simulink model "controller"  (R2015b)
settings: Solver=FixedStepAuto  StartTime=0.0  StopTime=50  FixedStep=0.01  RelTol=1e-3
values from neighbouring files (symbols this model uses):
  aGravityCompensation = 3.5837    [controllerParams.m]
  bGravityCompensation = 2.042    [controllerParams.m]
  cGravityCompensation = 0.3    [controllerParams.m]
  D2R = pi/180.0    (= 0.0174532925199)    [controllerParams.m]
  filterCoeffs = filterCoeffs.b    [controllerParams.m]
  K_CABLE = 3    [controllerParams.m]
  K_DAQ = 10    [controllerParams.m]
  KdElev = 0    [controllerParams.m]
  KdElevRate = 0.5    [controllerParams.m]
  KdPitch = 0.3    [controllerParams.m]
  KdPitchRate = 0.2    [controllerParams.m]
  KdTrav = 0    [controllerParams.m]
  KdTravRate = 0    [controllerParams.m]
  KE_C2D = -360/4096    (= -0.087890625)    [controllerParams.m]
  KiElev = 0    [controllerParams.m]
  KiElevRate = 0.2    [controllerParams.m]
  KiPitch = 0    [controllerParams.m]
  KiPitchRate = 0.2    [controllerParams.m]
  KiTrav = 0    [controllerParams.m]
  KiTravRate = 0    [controllerParams.m]
  KpElev = 0.76    [controllerParams.m]
  KpElevRate = 5.99    [controllerParams.m]
  KpPitch = 1.11    [controllerParams.m]
  KpPitchRate = 0.78    [controllerParams.m]
  KpTrav = 0.42    [controllerParams.m]
  KpTravRate = 2.49    [controllerParams.m]
  maxDeltaForce = 0.5    [controllerParams.m]
  maxElevCombForce = 2    [controllerParams.m]
  maxElevForce = 2    [controllerParams.m]
  maxElevRate = deg2rad(20)    [controllerParams.m]
  maxIntegralElev = inf    [controllerParams.m]
  maxIntegralElevRate = inf    [controllerParams.m]
  maxIntegralPitch = inf    [controllerParams.m]
  maxIntegralPitchRate = inf    [controllerParams.m]
  maxIntegralTrav = inf    [controllerParams.m]
  maxIntegralTravRate = inf    [controllerParams.m]
  maxPitchRate = deg2rad(35)    [controllerParams.m]
  maxTravForce = 0.9    [controllerParams.m]
  maxTravRate = deg2rad(20)    [controllerParams.m]
  minDeltaForce = -0.5    [controllerParams.m]
  minElevCombForce = 0    [controllerParams.m]
  minElevForce = -2    [controllerParams.m]
  minElevRate = -deg2rad(20)    [controllerParams.m]
  minIntegralElev = -inf    [controllerParams.m]
  minIntegralElevRate = -inf    [controllerParams.m]
  minIntegralPitch = -inf    [controllerParams.m]
  minIntegralPitchRate = -inf    [controllerParams.m]
  minIntegralTrav = -inf    [controllerParams.m]
  minIntegralTravRate = -inf    [controllerParams.m]
  minPitchRate = -deg2rad(35)    [controllerParams.m]
  minTravForce = -0.9    [controllerParams.m]
  minTravRate = -deg2rad(20)    [controllerParams.m]
  tuningElevRateRef = maxElevRate    [controllerParams.m]
  tuningElevRef = deg2rad(24.5)    [controllerParams.m]
  tuningPitchRateRef = maxPitchRate    [controllerParams.m]
  tuningPitchRef = deg2rad(30)    [controllerParams.m]
  tuningTravRateRef = maxTravRate    [controllerParams.m]
  tuningTravRef = deg2rad(45)    [controllerParams.m]
  VSUM_MAX = 30    [controllerParams.m]
undefined symbols (not defined in the file or in its folder): HIL
libraries: quarc_library x6, simulink_extras x2
settings Model: SimulationMode=external  ExtModeTrigDuration=10000  Creator=AER509  LastModifiedBy=kikut
settings SolverCC: PositivePriorityOrder=on
settings RTWCC: SystemTargetFile=quarc_win64.tlc  TemplateMakefile=quarc_default_tmf  Description=QUARC Win64 Target
settings STFCustomTargetCC: GeneratePreprocessorConditionals=Use local settings  CPPClassGenCompliant=off
settings GRTTargetCC: ParMdlRefBuildCompliant=off  CompOptLevelCompliant=off  CombineOutputUpdateFcns=off  MatFileLogging=off  CPPClassGenCompliant=off  GRTInterface=on  UseToolchainInfoCompliant=off  ExtMode=on  ExtModeMexFile=quarc_comm

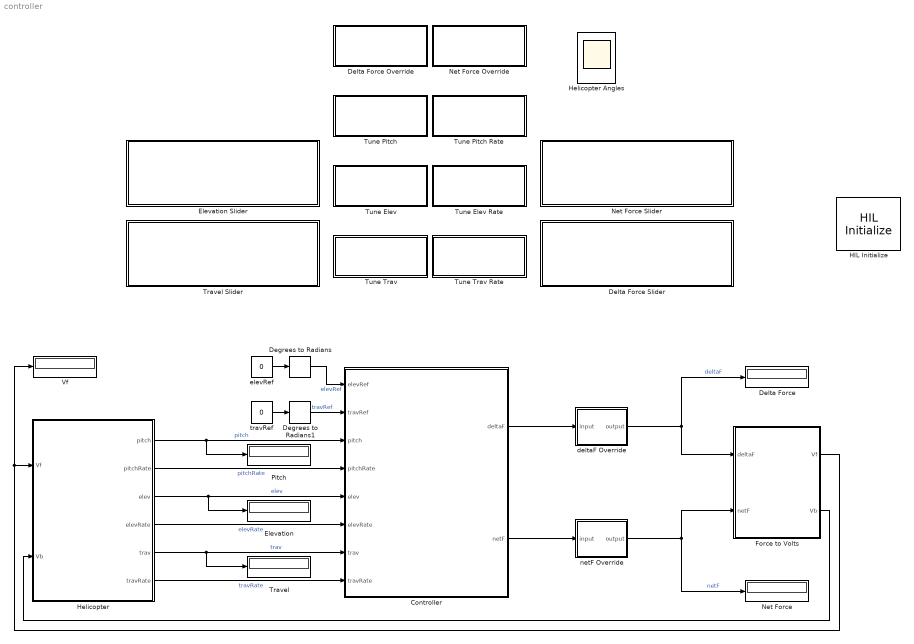
== system controller ==
  Controller : Subsystem
  Degrees to Radians : simulink_extras/Transformations/Degrees to Radians
  Degrees to Radians1 : simulink_extras/Transformations/Degrees to Radians
  Delta Force : Display
      settings: Decimation=2
  Delta Force Override : Subsystem  DialogController=hmiCreateDDGDialog  IsWebBlock=on  mask(MWDashboardBlock){webBlockId=4af075b6-758d-4f73-8e94-205a8f4b4bc9, webBlockType=sliderswitch, ShowInLibBrowser=on, ShowInitialText=on, HMISrcModelName=controller}
      mask prompts: webBlockId "WebBlock Id"; webBlockType "WebBlock Type"; HMISrcModelName "Source Model"
      mask Help: helpview([docroot '/mapfiles/simulink.map'], 'hmi_slider_switch')
      mask Display:
      | if strcmp(get_param(bdroot(gcb),'BlockDiagramType'), 'library')
      |     image([(matlabroot) '/toolbox/simulink/hmi/icons/SliderSwitch.png']);
      | end
  Delta Force Slider : Subsystem  DialogController=hmiCreateDDGDialog  IsWebBlock=on  mask(MWDashboardBlock){webBlockId=28de445a-717c-4887-bbc9-b4fa61ddbf15, webBlockType=slider, ShowInLibBrowser=on, ShowInitialText=on, HMISrcModelName=controller}
      mask prompts: webBlockId "WebBlock Id"; webBlockType "WebBlock Type"; HMISrcModelName "Source Model"
      mask Help: helpview([docroot '/mapfiles/simulink.map'], 'hmi_slider')
      mask Display:
      | if strcmp(get_param(bdroot(gcb),'BlockDiagramType'), 'library')
      |     image([(matlabroot) '/toolbox/simulink/hmi/icons/Slider.png']);
      | end
  Elevation : Display
      settings: Decimation=2
  Elevation Slider : Subsystem  DialogController=hmiCreateDDGDialog  IsWebBlock=on  mask(MWDashboardBlock){webBlockId=3dc72f43-562a-447e-a206-2819fa9ff394, webBlockType=slider, ShowInLibBrowser=on, ShowInitialText=on, HMISrcModelName=controller}
      mask prompts: webBlockId "WebBlock Id"; webBlockType "WebBlock Type"; HMISrcModelName "Source Model"
      mask Help: helpview([docroot '/mapfiles/simulink.map'], 'hmi_slider')
      mask Display:
      | if strcmp(get_param(bdroot(gcb),'BlockDiagramType'), 'library')
      |     image([(matlabroot) '/toolbox/simulink/hmi/icons/Slider.png']);
      | end
  Force to Volts : Subsystem
  HIL Initialize : quarc_library/Data Acquisition/Generic/Configuration/HIL Initialize  Priority=-99  object_name=HIL-1  board_type=q4  board_number=0  board_options=""  exclusive=off  active=off  hardware_clocks=[0:1]  clock_modes=[0 0]  initial_clock_frequencies=[]  set_clock_params_at_start=on  set_clock_params_at_switch_in=off  set_clock_frequencies_at_start=off  set_clock_frequencies_at_switch_in=off  analog_input_channels=[0:3]  analog_input_maximums=10  analog_input_minimums=-10  set_analog_input_params_at_start=off  set_analog_input_params_at_switch_in=off  analog_output_channels=[0:3]  analog_output_maximums=[10]  analog_output_minimums=[-10]  initial_analog_outputs=[0]  final_analog_outputs=[0]  watchdog_analog_outputs=0  set_analog_output_params_at_start=on  set_analog_output_params_at_switch_in=off  set_analog_outputs_at_start=on  set_analog_outputs_at_switch_in=off  set_analog_outputs_at_terminate=on  set_analog_outputs_at_switch_out=off  set_analog_outputs_on_watchdog=off  digital_input_channels=[]  digital_output_channels=[]  digital_output_configuration=[]  initial_digital_outputs=[1]  final_digital_outputs=[1]  watchdog_digital_outputs=[2]  set_digital_output_params_at_start=off  set_digital_output_params_at_switch_in=off  set_digital_outputs_at_start=on  set_digital_outputs_at_switch_in=off  set_digital_outputs_at_terminate=on  set_digital_outputs_at_switch_out=off  set_digital_outputs_on_watchdog=off  encoder_channels=[0:3]  quadrature=[4]  encoder_filter_frequency=(1/60e-9)/1  initial_encoder_counts=[0]  set_encoder_params_at_start=on  set_encoder_params_at_switch_in=off  set_encoder_counts_at_start=on  set_encoder_counts_at_switch_in=off  pwm_channels=[]  pwm_modes=[0]  pwm_frequency=(1/60e-9)/1024  pwm_configuration=[]  pwm_alignment=[]  pwm_polarity=[]  pwm_leading_deadband=[]  pwm_trailing_deadband=[]  initial_pwm_outputs=[0]  final_pwm_outputs=[0]  watchdog_pwm_outputs=[]  set_pwm_params_at_start=on  set_pwm_params_at_switch_in=off  set_pwm_outputs_at_start=on  set_pwm_outputs_at_switch_in=off  set_pwm_outputs_at_terminate=on  set_pwm_outputs_at_switch_out=off  set_pwm_outputs_on_watchdog=off  other_output_channels=[]  initial_other_outputs=[]  final_other_outputs=[]  watchdog_other_outputs=[]  set_other_outputs_at_start=off  set_other_outputs_at_switch_in=off  set_other_outputs_at_terminate=off  set_other_outputs_at_switch_out=off  set_other_outputs_on_watchdog=off
  Helicopter : Subsystem
  Helicopter Angles : Scope
      settings: Floating=on
  Net Force : Display
      settings: Decimation=2
  Net Force Override : Subsystem  DialogController=hmiCreateDDGDialog  IsWebBlock=on  mask(MWDashboardBlock){webBlockId=fdba1945-908f-46ed-bc95-797a072fabde, webBlockType=sliderswitch, ShowInLibBrowser=on, ShowInitialText=on, HMISrcModelName=controller}
      mask prompts: webBlockId "WebBlock Id"; webBlockType "WebBlock Type"; HMISrcModelName "Source Model"
      mask Help: helpview([docroot '/mapfiles/simulink.map'], 'hmi_slider_switch')
      mask Display:
      | if strcmp(get_param(bdroot(gcb),'BlockDiagramType'), 'library')
      |     image([(matlabroot) '/toolbox/simulink/hmi/icons/SliderSwitch.png']);
      | end
  Net Force Slider : Subsystem  DialogController=hmiCreateDDGDialog  IsWebBlock=on  mask(MWDashboardBlock){webBlockId=5aa08be6-65a4-4742-946a-0d5b8d80040d, webBlockType=slider, ShowInLibBrowser=on, ShowInitialText=on, HMISrcModelName=controller}
      mask prompts: webBlockId "WebBlock Id"; webBlockType "WebBlock Type"; HMISrcModelName "Source Model"
      mask Help: helpview([docroot '/mapfiles/simulink.map'], 'hmi_slider')
      mask Display:
      | if strcmp(get_param(bdroot(gcb),'BlockDiagramType'), 'library')
      |     image([(matlabroot) '/toolbox/simulink/hmi/icons/Slider.png']);
      | end
  Pitch : Display
      settings: Decimation=2
  Travel : Display
      settings: Decimation=2
  Travel Slider : Subsystem  DialogController=hmiCreateDDGDialog  IsWebBlock=on  mask(MWDashboardBlock){webBlockId=229cecbd-6c7e-45e2-a8fb-f334730ec9ad, webBlockType=slider, ShowInLibBrowser=on, ShowInitialText=on, HMISrcModelName=controller}
      mask prompts: webBlockId "WebBlock Id"; webBlockType "WebBlock Type"; HMISrcModelName "Source Model"
      mask Help: helpview([docroot '/mapfiles/simulink.map'], 'hmi_slider')
      mask Display:
      | if strcmp(get_param(bdroot(gcb),'BlockDiagramType'), 'library')
      |     image([(matlabroot) '/toolbox/simulink/hmi/icons/Slider.png']);
      | end
  Tune Elev : Subsystem  DialogController=hmiCreateDDGDialog  IsWebBlock=on  mask(MWDashboardBlock){webBlockId=e4a3f78e-3c07-4c1a-9f36-b612ed18eb99, webBlockType=sliderswitch, ShowInLibBrowser=on, ShowInitialText=on, HMISrcModelName=controller}
      mask prompts: webBlockId "WebBlock Id"; webBlockType "WebBlock Type"; HMISrcModelName "Source Model"
      mask Help: helpview([docroot '/mapfiles/simulink.map'], 'hmi_slider_switch')
      mask Display:
      | if strcmp(get_param(bdroot(gcb),'BlockDiagramType'), 'library')
      |     image([(matlabroot) '/toolbox/simulink/hmi/icons/SliderSwitch.png']);
      | end
  Tune Elev Rate : Subsystem  DialogController=hmiCreateDDGDialog  IsWebBlock=on  mask(MWDashboardBlock){webBlockId=5ad47bd1-198b-4ce9-a72d-63eab8823736, webBlockType=sliderswitch, ShowInLibBrowser=on, ShowInitialText=on, HMISrcModelName=controller}
      mask prompts: webBlockId "WebBlock Id"; webBlockType "WebBlock Type"; HMISrcModelName "Source Model"
      mask Help: helpview([docroot '/mapfiles/simulink.map'], 'hmi_slider_switch')
      mask Display:
      | if strcmp(get_param(bdroot(gcb),'BlockDiagramType'), 'library')
      |     image([(matlabroot) '/toolbox/simulink/hmi/icons/SliderSwitch.png']);
      | end
  Tune Pitch : Subsystem  DialogController=hmiCreateDDGDialog  IsWebBlock=on  mask(MWDashboardBlock){webBlockId=75521f76-8e1d-4ba6-a9fe-27f99e38a80e, webBlockType=sliderswitch, ShowInLibBrowser=on, ShowInitialText=on, HMISrcModelName=controller}
      mask prompts: webBlockId "WebBlock Id"; webBlockType "WebBlock Type"; HMISrcModelName "Source Model"
      mask Help: helpview([docroot '/mapfiles/simulink.map'], 'hmi_slider_switch')
      mask Display:
      | if strcmp(get_param(bdroot(gcb),'BlockDiagramType'), 'library')
      |     image([(matlabroot) '/toolbox/simulink/hmi/icons/SliderSwitch.png']);
      | end
  Tune Pitch Rate : Subsystem  DialogController=hmiCreateDDGDialog  IsWebBlock=on  mask(MWDashboardBlock){webBlockId=8d4346d9-8b28-4eb4-a156-b2d2519f8294, webBlockType=sliderswitch, ShowInLibBrowser=on, ShowInitialText=on, HMISrcModelName=controller}
      mask prompts: webBlockId "WebBlock Id"; webBlockType "WebBlock Type"; HMISrcModelName "Source Model"
      mask Help: helpview([docroot '/mapfiles/simulink.map'], 'hmi_slider_switch')
      mask Display:
      | if strcmp(get_param(bdroot(gcb),'BlockDiagramType'), 'library')
      |     image([(matlabroot) '/toolbox/simulink/hmi/icons/SliderSwitch.png']);
      | end
  Tune Trav : Subsystem  DialogController=hmiCreateDDGDialog  IsWebBlock=on  mask(MWDashboardBlock){webBlockId=cd129c28-8443-4f24-80a9-9a0e47c4c0a7, webBlockType=sliderswitch, ShowInLibBrowser=on, ShowInitialText=on, HMISrcModelName=controller}
      mask prompts: webBlockId "WebBlock Id"; webBlockType "WebBlock Type"; HMISrcModelName "Source Model"
      mask Help: helpview([docroot '/mapfiles/simulink.map'], 'hmi_slider_switch')
      mask Display:
      | if strcmp(get_param(bdroot(gcb),'BlockDiagramType'), 'library')
      |     image([(matlabroot) '/toolbox/simulink/hmi/icons/SliderSwitch.png']);
      | end
  Tune Trav Rate : Subsystem  DialogController=hmiCreateDDGDialog  IsWebBlock=on  mask(MWDashboardBlock){webBlockId=cd69dbce-f23b-4e1a-b675-1ecb4e30d85c, webBlockType=sliderswitch, ShowInLibBrowser=on, ShowInitialText=on, HMISrcModelName=controller}
      mask prompts: webBlockId "WebBlock Id"; webBlockType "WebBlock Type"; HMISrcModelName "Source Model"
      mask Help: helpview([docroot '/mapfiles/simulink.map'], 'hmi_slider_switch')
      mask Display:
      | if strcmp(get_param(bdroot(gcb),'BlockDiagramType'), 'library')
      |     image([(matlabroot) '/toolbox/simulink/hmi/icons/SliderSwitch.png']);
      | end
  Vf : Display
      settings: Decimation=2
  deltaF Override : Subsystem
  elevRef : Constant  Value=0
  netF Override : Subsystem
  travRef : Constant  Value=0
  wires:
  Helicopter/1(pitch) -> Pitch/1, Controller/3(pitch)  "pitch"
  Helicopter/2(pitchRate) -> Controller/4(pitchRate)  "pitchRate"
  Helicopter/3(elev) -> Elevation/1, Controller/5(elev)  "elev"
  Helicopter/4(elevRate) -> Controller/6(elevRate)  "elevRate"
  Helicopter/5(trav) -> Travel/1, Controller/7(trav)  "trav"
  Helicopter/6(travRate) -> Controller/8(travRate)  "travRate"
  Controller/2(netF) -> netF Override/1(input)
  netF Override/1(output) -> Net Force/1, Force to Volts/2(netF)  "netF"
  Controller/1(deltaF) -> deltaF Override/1(input)
  deltaF Override/1(output) -> Delta Force/1, Force to Volts/1(deltaF)  "deltaF"
  elevRef/1 -> Degrees to Radians/1
  travRef/1 -> Degrees to Radians1/1
  Degrees to Radians/1 -> Controller/1(elevRef)  "elevRef"
  Degrees to Radians1/1 -> Controller/2(travRef)  "travRef"
  Force to Volts/2(Vb) -> Helicopter/2(Vb)
  Force to Volts/1(Vf) -> Vf/1, Helicopter/1(Vf)

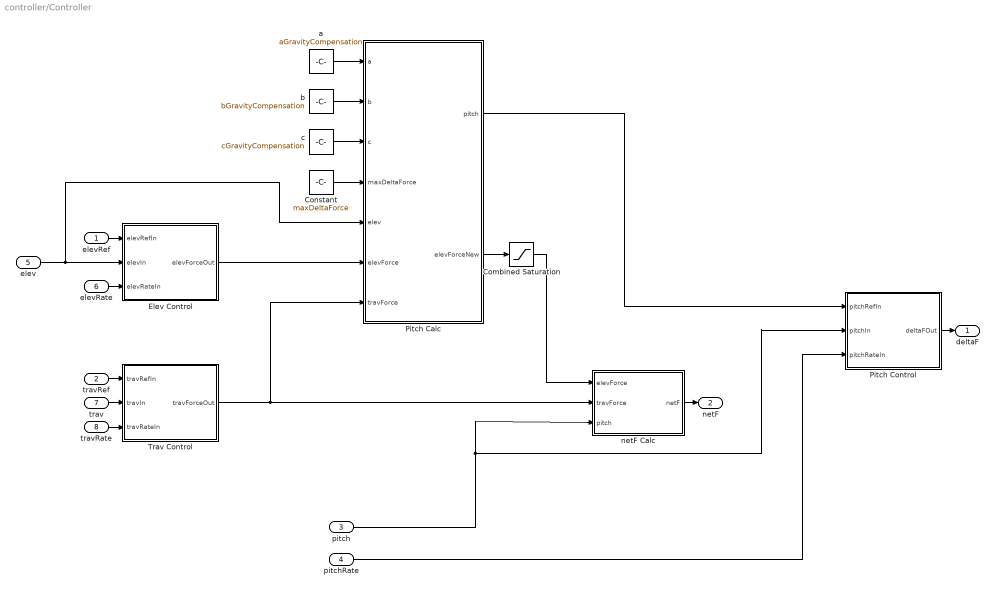
== system controller/Controller ==
  elevRef : Inport
  travRef : Inport  Port=2
  pitch : Inport  Port=3
  pitchRate : Inport  Port=4
  elev : Inport  Port=5
  elevRate : Inport  Port=6
  trav : Inport  Port=7
  travRate : Inport  Port=8
  Combined Saturation : Saturate  UpperLimit=maxElevCombForce  LowerLimit=minElevCombForce
  Constant : Constant  Value=maxDeltaForce
  Elev Control : Subsystem
  Pitch Calc : MATLAB Function  TreatAsAtomicUnit=on
  Pitch Control : Subsystem
  Trav Control : Subsystem
  a : Constant  Value=aGravityCompensation
  b : Constant  Value=bGravityCompensation
  c : Constant  Value=cGravityCompensation
  netF Calc : MATLAB Function  TreatAsAtomicUnit=on
  deltaF : Outport
  netF : Outport  Port=2
  wires:
  Trav Control/1(travForceOut) -> Pitch Calc/7(travForce), netF Calc/2(travForce)
  Elev Control/1(elevForceOut) -> Pitch Calc/6(elevForce)
  pitchRate/1 -> Pitch Control/3(pitchRateIn)
  netF Calc/1(netF) -> netF/1
  elev/1 -> Pitch Calc/5(elev), Elev Control/2(elevIn)
  elevRate/1 -> Elev Control/3(elevRateIn)
  elevRef/1 -> Elev Control/1(elevRefIn)
  Pitch Control/1(deltaFOut) -> deltaF/1
  Pitch Calc/2(elevForceNew) -> Combined Saturation/1
  travRate/1 -> Trav Control/3(travRateIn)
  trav/1 -> Trav Control/2(travIn)
  travRef/1 -> Trav Control/1(travRefIn)
  Pitch Calc/1(pitch) -> Pitch Control/1(pitchRefIn)
  pitch/1 -> netF Calc/3(pitch), Pitch Control/2(pitchIn)
  Constant/1 -> Pitch Calc/4(maxDeltaForce)
  Combined Saturation/1 -> netF Calc/1(elevForce)
  a/1 -> Pitch Calc/1(a)
  b/1 -> Pitch Calc/2(b)
  c/1 -> Pitch Calc/3(c)

== system controller/Delta Force Override ==

== system controller/Delta Force Slider ==

== system controller/Elevation Slider ==

== system controller/Force to Volts ==
  deltaF : Inport
  netF : Inport  Port=2
  Force Mixer : MATLAB Function  TreatAsAtomicUnit=on
  Force to Volt_Back : MATLAB Function  TreatAsAtomicUnit=on
  Force to Volt_Front : MATLAB Function  TreatAsAtomicUnit=on
  Vf : Outport
  Vb : Outport  Port=2
  wires:
  Force Mixer/1(F_f) -> Force to Volt_Front/1(F)
  Force to Volt_Front/1(V) -> Vf/1  "V_f"
  Force Mixer/2(F_b) -> Force to Volt_Back/1(F)
  Force to Volt_Back/1(V) -> Vb/1  "V_b"
  netF/1 -> Force Mixer/2(F)
  deltaF/1 -> Force Mixer/1(delta_F)

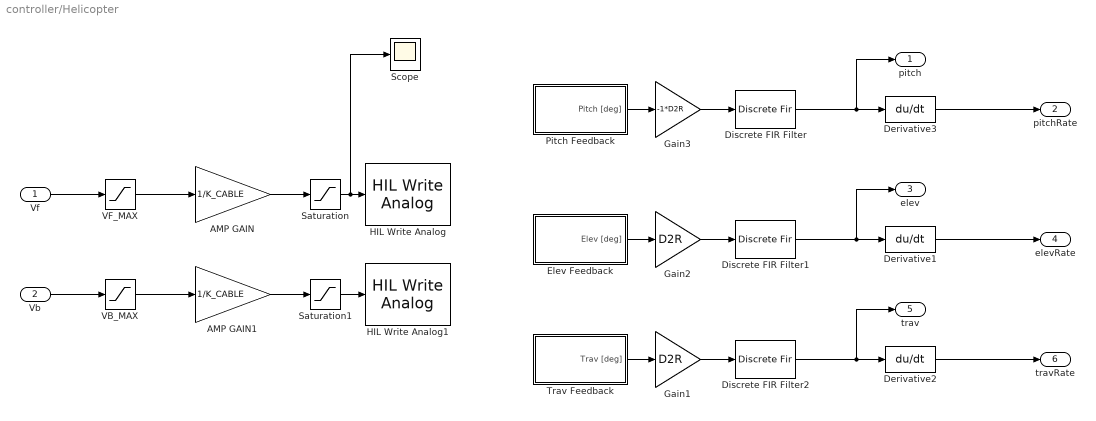
== system controller/Helicopter ==
  Vf : Inport
  Vb : Inport  Port=2
  AMP GAIN : Gain  Gain=1/K_CABLE
  AMP GAIN1 : Gain  Gain=1/K_CABLE
  Derivative1 : Derivative
  Derivative2 : Derivative
  Derivative3 : Derivative
  Discrete FIR Filter : DiscreteFir  Coefficients=filterCoeffs
  Discrete FIR Filter1 : DiscreteFir  Coefficients=filterCoeffs
  Discrete FIR Filter2 : DiscreteFir  Coefficients=filterCoeffs
  Elev Feedback : Subsystem
  Gain1 : Gain  Gain=D2R
  Gain2 : Gain  Gain=D2R
  Gain3 : Gain  Gain=-1*D2R
  HIL Write Analog : quarc_library/Data Acquisition/Generic/Immediate I//O/HIL Write Analog  object_name=HIL-1  channels=2  sample_time=-1  active=off  vector_input=off
  HIL Write Analog1 : quarc_library/Data Acquisition/Generic/Immediate I//O/HIL Write Analog  object_name=HIL-1  channels=3  sample_time=-1  active=off  vector_input=off
  Pitch Feedback : Subsystem
  Saturation : Saturate  UpperLimit=K_DAQ*0.5  LowerLimit=-K_DAQ*0.5
  Saturation1 : Saturate  UpperLimit=K_DAQ*0.5  LowerLimit=-K_DAQ*0.5
  Scope : Scope
  Trav Feedback : Subsystem
  VB_MAX : Saturate  UpperLimit=VSUM_MAX*0.5  LowerLimit=-VSUM_MAX*0.5
  VF_MAX : Saturate  UpperLimit=VSUM_MAX*0.5  LowerLimit=-VSUM_MAX*0.5  LinearizeAsGain=off
  pitch : Outport
  pitchRate : Outport  Port=2
  elev : Outport  Port=3
  elevRate : Outport  Port=4
  trav : Outport  Port=5
  travRate : Outport  Port=6
  wires:
  VB_MAX/1 -> AMP GAIN1/1
  Pitch Feedback/1(Pitch [deg]) -> Gain3/1
  Trav Feedback/1(Trav [deg]) -> Gain1/1
  Gain3/1 -> Discrete FIR Filter/1
  Saturation/1 -> Scope/1, HIL Write Analog/1
  Vf/1 -> VF_MAX/1
  VF_MAX/1 -> AMP GAIN/1
  AMP GAIN/1 -> Saturation/1
  Saturation1/1 -> HIL Write Analog1/1
  Discrete FIR Filter/1 -> pitch/1, Derivative3/1
  AMP GAIN1/1 -> Saturation1/1
  Elev Feedback/1(Elev [deg]) -> Gain2/1
  Vb/1 -> VB_MAX/1
  Derivative3/1 -> pitchRate/1
  Gain2/1 -> Discrete FIR Filter1/1
  Discrete FIR Filter1/1 -> elev/1, Derivative1/1
  Derivative1/1 -> elevRate/1
  Gain1/1 -> Discrete FIR Filter2/1
  Discrete FIR Filter2/1 -> trav/1, Derivative2/1
  Derivative2/1 -> travRate/1

== system controller/Net Force Override ==

== system controller/Net Force Slider ==

== system controller/Travel Slider ==

== system controller/Tune Elev ==

== system controller/Tune Elev Rate ==

== system controller/Tune Pitch ==

== system controller/Tune Pitch Rate ==

== system controller/Tune Trav ==

== system controller/Tune Trav Rate ==

== system controller/deltaF Override ==
  input : Inport
  Tune Selector : Subsystem
  tuneRef : Constant  Value=0
  output : Outport
  wires:
  tuneRef/1 -> Tune Selector/1(tuneRef)
  input/1 -> Tune Selector/2(defaultRef)
  Tune Selector/1("output ") -> output/1

== system controller/netF Override ==
  input : Inport
  Tune Selector : Subsystem
  tuneRef : Constant  Value=0.5875
  output : Outport
  wires:
  tuneRef/1 -> Tune Selector/1(tuneRef)
  input/1 -> Tune Selector/2(defaultRef)
  Tune Selector/1("output ") -> output/1

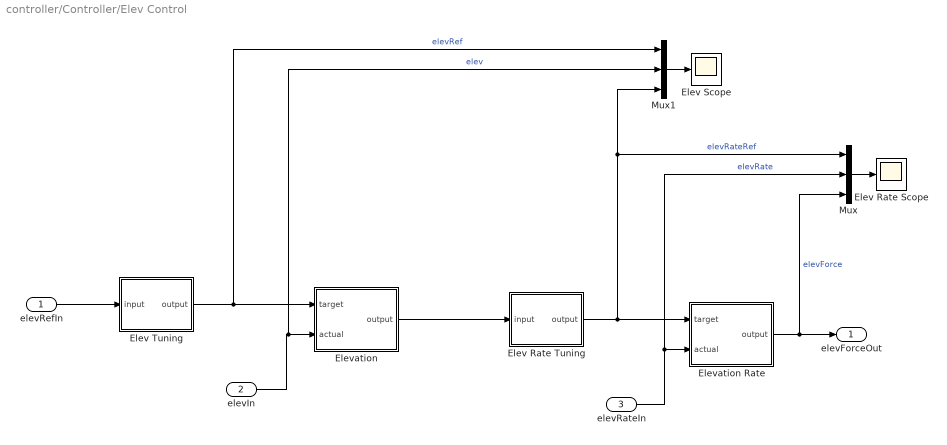
== system controller/Controller/Elev Control ==
  elevRefIn : Inport
  elevIn : Inport  Port=2
  elevRateIn : Inport  Port=3
  Elev Rate Scope : Scope
  Elev Rate Tuning : Subsystem
  Elev Scope : Scope
  Elev Tuning : Subsystem
  Elevation : Subsystem
  Elevation Rate : Subsystem
  Mux : Mux  Inputs=3
  Mux1 : Mux  Inputs=3
  elevForceOut : Outport
  wires:
  Elev Tuning/1(output) -> Mux1/1, Elevation/1(target)  "elevRef"
  Elev Rate Tuning/1(output) -> Mux1/3, Mux/1, Elevation Rate/1(target)  "elevRateRef"
  Elevation/1(output) -> Elev Rate Tuning/1(input)
  Elevation Rate/1(output) -> Mux/3, elevForceOut/1  "elevForce"
  elevRefIn/1 -> Elev Tuning/1(input)
  elevIn/1 -> Mux1/2, Elevation/2(actual)  "elev"
  elevRateIn/1 -> Mux/2, Elevation Rate/2(actual)  "elevRate"
  Mux/1 -> Elev Rate Scope/1
  Mux1/1 -> Elev Scope/1

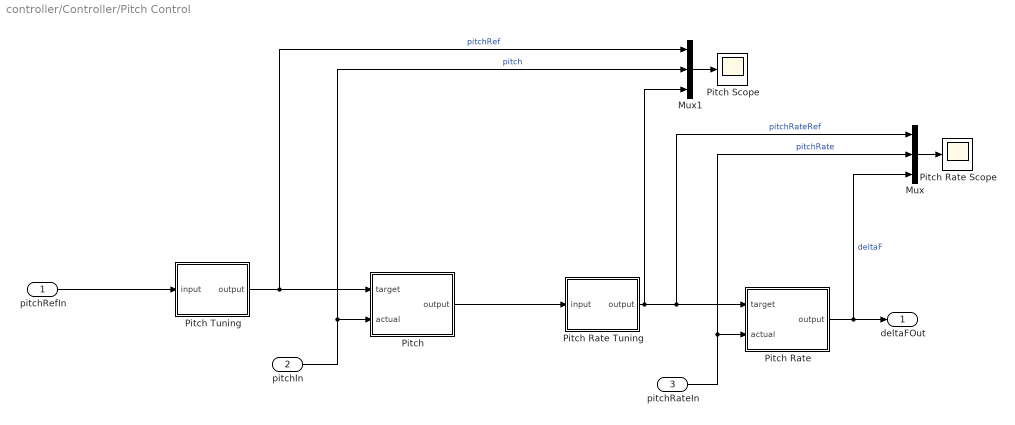
== system controller/Controller/Pitch Control ==
  pitchRefIn : Inport
  pitchIn : Inport  Port=2
  pitchRateIn : Inport  Port=3
  Mux : Mux  Inputs=3
  Mux1 : Mux  Inputs=3
  Pitch : Subsystem
  Pitch Rate : Subsystem
  Pitch Rate Scope : Scope
  Pitch Rate Tuning : Subsystem
  Pitch Scope : Scope
  Pitch Tuning : Subsystem
  deltaFOut : Outport
  wires:
  Pitch Rate/1(output) -> Mux/3, deltaFOut/1  "deltaF"
  pitchIn/1 -> Mux1/2, Pitch/2(actual)  "pitch"
  pitchRefIn/1 -> Pitch Tuning/1(input)
  Pitch Rate Tuning/1(output) -> Mux1/3, Mux/1, Pitch Rate/1(target)  "pitchRateRef"
  Pitch Tuning/1(output) -> Mux1/1, Pitch/1(target)  "pitchRef"
  Pitch/1(output) -> Pitch Rate Tuning/1(input)
  pitchRateIn/1 -> Mux/2, Pitch Rate/2(actual)  "pitchRate"
  Mux/1 -> Pitch Rate Scope/1
  Mux1/1 -> Pitch Scope/1

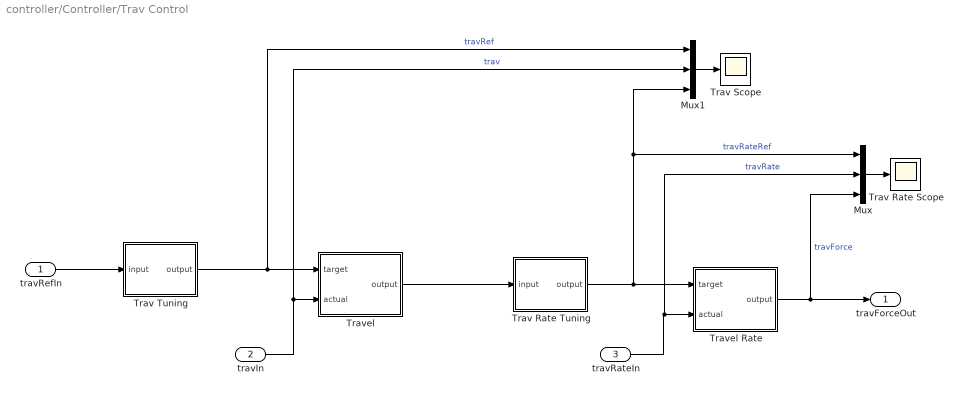
== system controller/Controller/Trav Control ==
  travRefIn : Inport
  travIn : Inport  Port=2
  travRateIn : Inport  Port=3
  Mux : Mux  Inputs=3
  Mux1 : Mux  Inputs=3
  Trav Rate Scope : Scope
  Trav Rate Tuning : Subsystem
  Trav Scope : Scope
  Trav Tuning : Subsystem
  Travel : Subsystem
  Travel Rate : Subsystem
  travForceOut : Outport
  wires:
  Travel Rate/1(output) -> Mux/3, travForceOut/1  "travForce"
  travRateIn/1 -> Mux/2, Travel Rate/2(actual)  "travRate"
  travIn/1 -> Mux1/2, Travel/2(actual)  "trav"
  travRefIn/1 -> Trav Tuning/1(input)
  Trav Tuning/1(output) -> Mux1/1, Travel/1(target)  "travRef"
  Travel/1(output) -> Trav Rate Tuning/1(input)
  Trav Rate Tuning/1(output) -> Mux1/3, Mux/1, Travel Rate/1(target)  "travRateRef"
  Mux/1 -> Trav Rate Scope/1
  Mux1/1 -> Trav Scope/1

== system controller/Helicopter/Elev Feedback ==
  Bias : Bias
  Count2Degree : Gain  Gain=KE_C2D
  HIL Read Encoder : quarc_library/Data Acquisition/Generic/Immediate I//O/HIL Read Encoder  object_name=HIL-1  channels=3  sample_time=qc_get_step_size  active=on  vector_output=off  data_type_mode=Inherit via back propagation  data_type=double
  Elev [deg] : Outport
  wires:
  Count2Degree/1 -> Bias/1
  Bias/1 -> Elev [deg]/1
  HIL Read Encoder/1 -> Count2Degree/1

== system controller/Helicopter/Pitch Feedback ==
  Bias : Bias
  Count2Degree : Gain  Gain=KE_C2D*0.5
  HIL Read Encoder : quarc_library/Data Acquisition/Generic/Immediate I//O/HIL Read Encoder  object_name=HIL-1  channels=2  sample_time=qc_get_step_size  active=on  vector_output=off  data_type_mode=Inherit via back propagation  data_type=double
  Pitch [deg] : Outport
  wires:
  Count2Degree/1 -> Bias/1
  Bias/1 -> Pitch [deg]/1
  HIL Read Encoder/1 -> Count2Degree/1

== system controller/Helicopter/Trav Feedback ==
  Bias : Bias
  Count2Degree : Gain  Gain=KE_C2D*0.5
  HIL Read Encoder : quarc_library/Data Acquisition/Generic/Immediate I//O/HIL Read Encoder  object_name=HIL-1  channels=1  sample_time=qc_get_step_size  active=on  vector_output=off  data_type_mode=Inherit via back propagation  data_type=double
  Trav [deg] : Outport
  wires:
  Count2Degree/1 -> Bias/1
  Bias/1 -> Trav [deg]/1
  HIL Read Encoder/1 -> Count2Degree/1

== system controller/deltaF Override/Tune Selector ==
  tuneRef : Inport
  defaultRef : Inport  Port=2
  Multiport Switch : MultiPortSwitch  DataPortOrder=Zero-based contiguous  Inputs=2
  deltaF : Constant  Value=0
  "output " : Outport
  wires:
  deltaF/1 -> Multiport Switch/1
  defaultRef/1 -> Multiport Switch/2
  Multiport Switch/1 -> "output "/1
  tuneRef/1 -> Multiport Switch/3

== system controller/netF Override/Tune Selector ==
  tuneRef : Inport
  defaultRef : Inport  Port=2
  Multiport Switch : MultiPortSwitch  DataPortOrder=Zero-based contiguous  Inputs=2  DataPortIndices={1,2}
  netF : Constant  Value=0
  "output " : Outport
  wires:
  netF/1 -> Multiport Switch/1
  defaultRef/1 -> Multiport Switch/2
  Multiport Switch/1 -> "output "/1
  tuneRef/1 -> Multiport Switch/3

== system controller/Controller/Elev Control/Elev Rate Tuning ==
  input : Inport
  Step : Step  Time=2  After=tuningElevRateRef  SampleTime=0
  Tune Selector : Subsystem
  output : Outport
  wires:
  Step/1 -> Tune Selector/1(tuneRef)
  input/1 -> Tune Selector/2(defaultRef)
  Tune Selector/1("output ") -> output/1

== system controller/Controller/Elev Control/Elev Tuning ==
  input : Inport
  Step : Step  Time=2  After=tuningElevRef  SampleTime=0
  Tune Selector : Subsystem
  output : Outport
  wires:
  Step/1 -> Tune Selector/1(tuneRef)
  input/1 -> Tune Selector/2(defaultRef)
  Tune Selector/1("output ") -> output/1

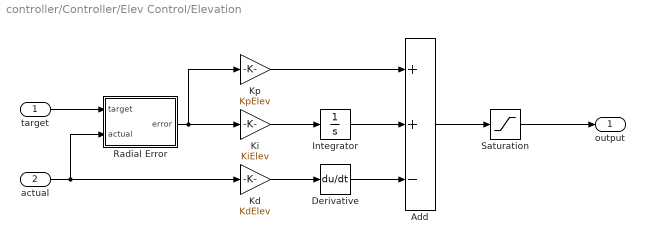
== system controller/Controller/Elev Control/Elevation ==
  target : Inport
  actual : Inport  Port=2
  Add : Sum  Inputs=++-
  Derivative : Derivative
  Integrator : Integrator  LimitOutput=on  UpperSaturationLimit=maxIntegralElev  LowerSaturationLimit=minIntegralElev
  Kd : Gain  Gain=KdElev
  Ki : Gain  Gain=KiElev
  Kp : Gain  Gain=KpElev
  Radial Error : MATLAB Function  TreatAsAtomicUnit=on
  Saturation : Saturate  UpperLimit=maxElevRate  LowerLimit=minElevRate
  output : Outport
  wires:
  Radial Error/1(error) -> Kp/1, Ki/1
  actual/1 -> Radial Error/2(actual), Kd/1
  Kd/1 -> Derivative/1
  Kp/1 -> Add/1
  Add/1 -> Saturation/1
  Integrator/1 -> Add/2
  target/1 -> Radial Error/1(target)
  Saturation/1 -> output/1
  Derivative/1 -> Add/3
  Ki/1 -> Integrator/1

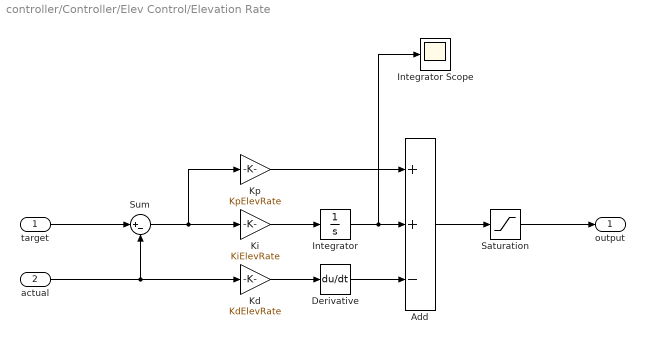
== system controller/Controller/Elev Control/Elevation Rate ==
  target : Inport
  actual : Inport  Port=2
  Add : Sum  Inputs=++-
  Derivative : Derivative
  Integrator : Integrator  LimitOutput=on  UpperSaturationLimit=maxIntegralElevRate  LowerSaturationLimit=minIntegralElevRate
  Integrator Scope : Scope
  Kd : Gain  Gain=KdElevRate
  Ki : Gain  Gain=KiElevRate
  Kp : Gain  Gain=KpElevRate
  Saturation : Saturate  UpperLimit=maxElevForce  LowerLimit=minElevForce
  Sum : Sum  Inputs=|+-
  output : Outport
  wires:
  Sum/1 -> Kp/1, Ki/1
  actual/1 -> Sum/2, Kd/1
  Kd/1 -> Derivative/1
  Kp/1 -> Add/1
  Add/1 -> Saturation/1
  Integrator/1 -> Integrator Scope/1, Add/2
  target/1 -> Sum/1
  Saturation/1 -> output/1
  Derivative/1 -> Add/3
  Ki/1 -> Integrator/1

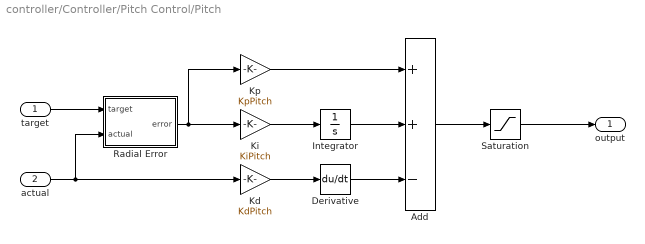
== system controller/Controller/Pitch Control/Pitch ==
  target : Inport
  actual : Inport  Port=2
  Add : Sum  Inputs=++-
  Derivative : Derivative
  Integrator : Integrator  LimitOutput=on  UpperSaturationLimit=maxIntegralPitch  LowerSaturationLimit=minIntegralPitch
  Kd : Gain  Gain=KdPitch
  Ki : Gain  Gain=KiPitch
  Kp : Gain  Gain=KpPitch
  Radial Error : MATLAB Function  TreatAsAtomicUnit=on
  Saturation : Saturate  UpperLimit=maxPitchRate  LowerLimit=minPitchRate
  output : Outport
  wires:
  Radial Error/1(error) -> Kp/1, Ki/1
  actual/1 -> Radial Error/2(actual), Kd/1
  Kd/1 -> Derivative/1
  Kp/1 -> Add/1
  Add/1 -> Saturation/1
  Integrator/1 -> Add/2
  target/1 -> Radial Error/1(target)
  Saturation/1 -> output/1
  Derivative/1 -> Add/3
  Ki/1 -> Integrator/1

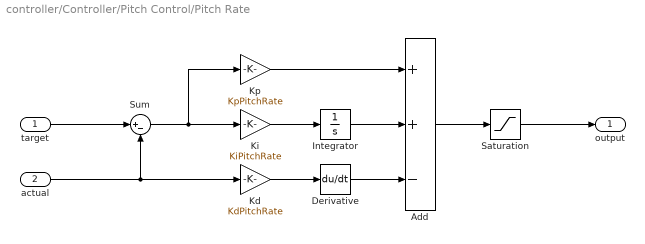
== system controller/Controller/Pitch Control/Pitch Rate ==
  target : Inport
  actual : Inport  Port=2
  Add : Sum  Inputs=++-
  Derivative : Derivative
  Integrator : Integrator  LimitOutput=on  UpperSaturationLimit=maxIntegralPitchRate  LowerSaturationLimit=minIntegralPitchRate
  Kd : Gain  Gain=KdPitchRate
  Ki : Gain  Gain=KiPitchRate
  Kp : Gain  Gain=KpPitchRate
  Saturation : Saturate  UpperLimit=maxDeltaForce  LowerLimit=minDeltaForce
  Sum : Sum  Inputs=|+-
  output : Outport
  wires:
  Sum/1 -> Kp/1, Ki/1
  actual/1 -> Sum/2, Kd/1
  Kd/1 -> Derivative/1
  Kp/1 -> Add/1
  Add/1 -> Saturation/1
  Integrator/1 -> Add/2
  target/1 -> Sum/1
  Saturation/1 -> output/1
  Derivative/1 -> Add/3
  Ki/1 -> Integrator/1

== system controller/Controller/Pitch Control/Pitch Rate Tuning ==
  input : Inport
  Step : Step  Time=2  After=tuningPitchRateRef  SampleTime=0
  Tune Selector : Subsystem
  output : Outport
  wires:
  Step/1 -> Tune Selector/1(tuneRef)
  input/1 -> Tune Selector/2(defaultRef)
  Tune Selector/1("output ") -> output/1

== system controller/Controller/Pitch Control/Pitch Tuning ==
  input : Inport
  Step : Step  Time=2  After=tuningPitchRef  SampleTime=0
  Tune Selector : Subsystem
  output : Outport
  wires:
  Step/1 -> Tune Selector/1(tuneRef)
  input/1 -> Tune Selector/2(defaultRef)
  Tune Selector/1("output ") -> output/1

== system controller/Controller/Trav Control/Trav Rate Tuning ==
  input : Inport
  Step : Step  Time=10  After=tuningTravRateRef  SampleTime=0
  Tune Selector : Subsystem
  output : Outport
  wires:
  Step/1 -> Tune Selector/1(tuneRef)
  input/1 -> Tune Selector/2(defaultRef)
  Tune Selector/1("output ") -> output/1

== system controller/Controller/Trav Control/Trav Tuning ==
  input : Inport
  Step : Step  Time=10  After=tuningTravRef  SampleTime=0
  Tune Selector : Subsystem
  output : Outport
  wires:
  Step/1 -> Tune Selector/1(tuneRef)
  input/1 -> Tune Selector/2(defaultRef)
  Tune Selector/1("output ") -> output/1

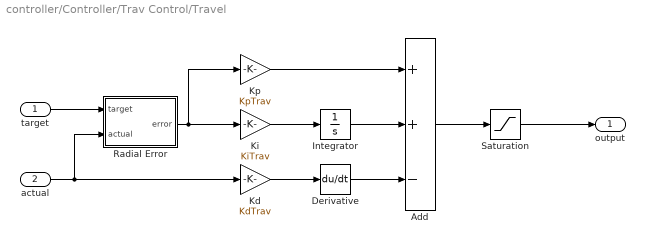
== system controller/Controller/Trav Control/Travel ==
  target : Inport
  actual : Inport  Port=2
  Add : Sum  Inputs=++-
  Derivative : Derivative
  Integrator : Integrator  LimitOutput=on  UpperSaturationLimit=maxIntegralTrav  LowerSaturationLimit=minIntegralTrav
  Kd : Gain  Gain=KdTrav
  Ki : Gain  Gain=KiTrav
  Kp : Gain  Gain=KpTrav
  Radial Error : MATLAB Function  TreatAsAtomicUnit=on
  Saturation : Saturate  UpperLimit=maxTravRate  LowerLimit=minTravRate
  output : Outport
  wires:
  Radial Error/1(error) -> Kp/1, Ki/1
  actual/1 -> Radial Error/2(actual), Kd/1
  Kd/1 -> Derivative/1
  Kp/1 -> Add/1
  Add/1 -> Saturation/1
  Integrator/1 -> Add/2
  target/1 -> Radial Error/1(target)
  Saturation/1 -> output/1
  Derivative/1 -> Add/3
  Ki/1 -> Integrator/1

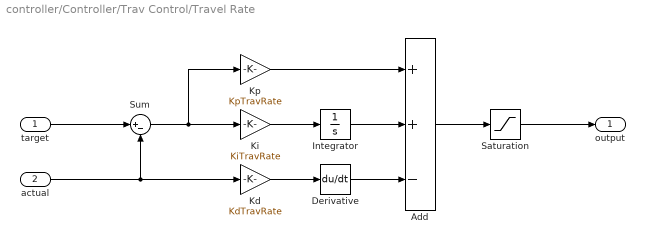
== system controller/Controller/Trav Control/Travel Rate ==
  target : Inport
  actual : Inport  Port=2
  Add : Sum  Inputs=++-
  Derivative : Derivative
  Integrator : Integrator  LimitOutput=on  UpperSaturationLimit=maxIntegralTravRate  LowerSaturationLimit=minIntegralTravRate
  Kd : Gain  Gain=KdTravRate
  Ki : Gain  Gain=KiTravRate
  Kp : Gain  Gain=KpTravRate
  Saturation : Saturate  UpperLimit=maxTravForce  LowerLimit=minTravForce
  Sum : Sum  Inputs=|+-
  output : Outport
  wires:
  Sum/1 -> Kp/1, Ki/1
  actual/1 -> Sum/2, Kd/1
  Kd/1 -> Derivative/1
  Kp/1 -> Add/1
  Add/1 -> Saturation/1
  Integrator/1 -> Add/2
  target/1 -> Sum/1
  Saturation/1 -> output/1
  Derivative/1 -> Add/3
  Ki/1 -> Integrator/1

== system controller/Controller/Elev Control/Elev Rate Tuning/Tune Selector ==
  tuneRef : Inport
  defaultRef : Inport  Port=2
  Multiport Switch : MultiPortSwitch  DataPortOrder=Zero-based contiguous  Inputs=2
  elevRate : Constant  Value=0
  "output " : Outport
  wires:
  elevRate/1 -> Multiport Switch/1
  defaultRef/1 -> Multiport Switch/2
  Multiport Switch/1 -> "output "/1
  tuneRef/1 -> Multiport Switch/3

== system controller/Controller/Elev Control/Elev Tuning/Tune Selector ==
  tuneRef : Inport
  defaultRef : Inport  Port=2
  Multiport Switch : MultiPortSwitch  DataPortOrder=Zero-based contiguous  Inputs=2
  elev : Constant
  "output " : Outport
  wires:
  elev/1 -> Multiport Switch/1
  defaultRef/1 -> Multiport Switch/2
  Multiport Switch/1 -> "output "/1
  tuneRef/1 -> Multiport Switch/3

== system controller/Controller/Pitch Control/Pitch Rate Tuning/Tune Selector ==
  tuneRef : Inport
  defaultRef : Inport  Port=2
  Multiport Switch : MultiPortSwitch  DataPortOrder=Zero-based contiguous  Inputs=2
  pitchRate : Constant  Value=0
  "output " : Outport
  wires:
  pitchRate/1 -> Multiport Switch/1
  defaultRef/1 -> Multiport Switch/2
  Multiport Switch/1 -> "output "/1
  tuneRef/1 -> Multiport Switch/3

== system controller/Controller/Pitch Control/Pitch Tuning/Tune Selector ==
  tuneRef : Inport
  defaultRef : Inport  Port=2
  Multiport Switch : MultiPortSwitch  DataPortOrder=Zero-based contiguous  Inputs=2
  pitch : Constant  Value=0
  "output " : Outport
  wires:
  pitch/1 -> Multiport Switch/1
  defaultRef/1 -> Multiport Switch/2
  Multiport Switch/1 -> "output "/1
  tuneRef/1 -> Multiport Switch/3

== system controller/Controller/Trav Control/Trav Rate Tuning/Tune Selector ==
  tuneRef : Inport
  defaultRef : Inport  Port=2
  Multiport Switch : MultiPortSwitch  DataPortOrder=Zero-based contiguous  Inputs=2
  travRate : Constant
  "output " : Outport
  wires:
  travRate/1 -> Multiport Switch/1
  defaultRef/1 -> Multiport Switch/2
  Multiport Switch/1 -> "output "/1
  tuneRef/1 -> Multiport Switch/3

== system controller/Controller/Trav Control/Trav Tuning/Tune Selector ==
  tuneRef : Inport
  defaultRef : Inport  Port=2
  Multiport Switch : MultiPortSwitch  DataPortOrder=Zero-based contiguous  Inputs=2
  trav : Constant  Value=0
  "output " : Outport
  wires:
  trav/1 -> Multiport Switch/1
  defaultRef/1 -> Multiport Switch/2
  Multiport Switch/1 -> "output "/1
  tuneRef/1 -> Multiport Switch/3

== matlab function controller/Force to Volts/Force Mixer ==
  data: delta_F input; F_f output; F input; F_b output
function [F_f, F_b] = fcn(delta_F, F)
    F_f = (F + delta_F) /2;
    F_b = (F - delta_F) /2;
end

== matlab function controller/Force to Volts/Force to Volt_Front ==
  data: F input; V output
function V = fcn(F)
    a = 0.0053;
    b = 0.0022;
    c = -abs(F);

    V = (-b + sqrt(b^2 - 4*a*c)) / (2*a);

    if F < 0
        V = -V;
    end
end

== matlab function controller/Force to Volts/Force to Volt_Back ==
  data: F input; V output
function V = fcn(F)
    a = 0.0053;
    b = 0.0022;
    c = -abs(F);

    V = (-b + sqrt(b^2 - 4*a*c)) / (2*a);

    if F < 0
        V = -V;
    end
end

== matlab function controller/Controller/Elev Control/Elevation/Radial Error ==
  data: target input; error output; actual input
function error = fcn(target, actual)
    % Find minimum angle between two angles
    error = target - actual;
    error = mod(error + pi, 2 * pi) - pi;
end

== matlab function controller/Controller/netF Calc ==
  data: netF output; elevForce input; travForce input; pitch input
function netF  = fcn(elevForce, travForce, pitch)
    if abs(pitch) >= pi / 2
        % Avoid division by zero when pitch is 90 or -90
        netF = abs(travForce);
    else
        netF = elevForce / cos(pitch);
    end
end

== matlab function controller/Controller/Pitch Calc ==
  data: a input; b input; c input; maxDeltaForce input; pitch output; elev input; elevForceNew output; elevForce input; travForce input
function [pitch, elevForceNew]  = fcn(a, b, c, maxDeltaForce, elev, elevForce, travForce)
    % Add feedforward compensator
    compForce = a * elev ^ 2 + b * elev + c;
    elevForce = elevForce + compForce;
    
    % Ensure elevForce is greater than or equal to zero
    if elevForce < 0
        elevForce = 0;
    end
    
    % Ensure force stays above minimum to maintain full deltaF
    if sqrt(elevForce ^ 2 + travForce ^ 2) < (maxDeltaForce / 2)
        elevForce = sqrt((maxDeltaForce / 2) ^ 2 - travForce ^ 2);
    end
    elevForceNew = elevForce;
    
    % Compute pitch angle
    pitch = atan2(travForce, elevForceNew);
end

== matlab function controller/Controller/Trav Control/Travel/Radial Error ==
  data: target input; error output; actual input
function error = fcn(target, actual)
    % Find minimum angle between two angles
    error = target - actual;
    error = mod(error + pi, 2 * pi) - pi;
end

== matlab function controller/Controller/Pitch Control/Pitch/Radial Error ==
  data: target input; error output; actual input
function error = fcn(target, actual)
    % Find minimum angle between two angles
    error = target - actual;
    error = mod(error + pi, 2 * pi) - pi;
end
